simulink subsystem "duty_cycle_allocation_mT_P_2"  (R2020b)
settings: Solver=VariableStepAuto  StartTime=0.0  StopTime=10.0  RelTol=1e-3
undefined symbols (not defined in the file): T_P_1, T_P_2
settings Model: Creator=leop9  LastModifiedBy=Previ

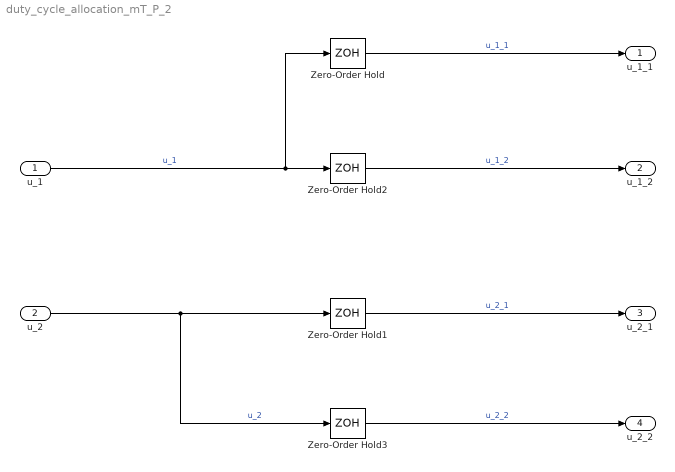
== system duty_cycle_allocation_mT_P_2 ==
  u_1 : Inport
  u_2 : Inport  Port=2
  Zero-Order Hold : ZeroOrderHold  SampleTime=T_P_1
  Zero-Order Hold1 : ZeroOrderHold  SampleTime=T_P_1
  Zero-Order Hold2 : ZeroOrderHold  SampleTime=T_P_2
  Zero-Order Hold3 : ZeroOrderHold  SampleTime=T_P_2
  u_1_1 : Outport
  u_1_2 : Outport  Port=2
  u_2_1 : Outport  Port=3
  u_2_2 : Outport  Port=4
  wires:
  u_1/1 -> Zero-Order Hold/1, Zero-Order Hold2/1  "u_1"
  u_2/1 -> Zero-Order Hold3/1, Zero-Order Hold1/1  "u_2"
  Zero-Order Hold2/1 -> u_1_2/1  "u_1_2"
  Zero-Order Hold/1 -> u_1_1/1  "u_1_1"
  Zero-Order Hold3/1 -> u_2_2/1  "u_2_2"
  Zero-Order Hold1/1 -> u_2_1/1  "u_2_1"
